simulink model "M_6DoF_BS_Full_backup_11_25_2018"  (R2018a)
settings: Solver=ode4  StartTime=0.0  StopTime=80  FixedStep=0.01  RelTol=1e-3  EnableMultiTasking=on
values from neighbouring files (symbols this model uses):
  b = 1.5652e-08 * (60/(2*pi))^2    (= 1.42729124973e-06)    [Main_run.m]    (also in golden_search.m = x2)
  cbar = 0.04    [Main_run.m]
  Cd = 0.001    [Main_run.m]
  deltaT = 15    [Main_run.m]
  g = 9.81    [Main_run.m]
  Gama1 = diag([3,3,3])    [Main_run.m]
  Gama2 = diag([0.1,0.1,0.1])    [Main_run.m]
  I_B = diag([Ix,Iy,Iz])    [Main_run.m]
  I_r = 3.357e-5    (= 3.357e-05)    [Main_run.m]
  InitialEulerAngles = [psi_i,theta_i,phi_i]    [Main_run.m]
  k = 2.0862e-10 * (60/(2*pi))^2    (= 1.90238627983e-08)    [Main_run.m]    (also in golden_search.m = 2)
  Kd = diag([2,2,2])    [Main_run.m]
  Ki = diag([0.01,0.01,0.01])    [Main_run.m]
  Kp = diag([1,1,1])    [Main_run.m]
  l = 0.225    [Main_run.m]    (also in try1.m = nb * trapz(psi, cl * 0.5 .* rho .* (vt*u).^2 .*c2 , 2) / (2*; try2.m = nb * trapz(psi, cl * 0.5 .* rho .* (vt*u).^2 .*c2 , 2) / (2*)
  Lambda = diag([10,10,10])    [Main_run.m]
  m = 1.035 * 4/6    (= 0.69)    [Main_run.m]
  Omega_i = [0;0;0]    [Main_run.m]
  r = linspace(floor(nr*0.01)/nr,1,nr)    [Main_run.m]    (also in Propeller.m = geometry(10,1:nr); try1.m = geometry(10,1:nr); try2.m = geometry(10,1:nr))
  R_i = [0.0;0.0;0.0]    [Main_run.m]
  t_phase3 = 10    [Main_run.m]
  Tbar = diag([15,15,15])    [Main_run.m]
  tf_phase1 = 10    [Main_run.m]
  tf_phase2 = tf_phase1 + length_phase2*60    (= 70)    [Main_run.m]
  V_i = [0.0;0.0;-0.001]    [Main_run.m]
  Wind_dir = 30 + 180    (= 210)    [Main_run.m]
  xdot_cruise = 15    [Main_run.m]
  zf_phase1 = -40    [Main_run.m]
undefined symbols (not defined in the file or in its folder): eul_0, HDBK, MIL, Moderate, wind_table, wind_time
libraries: sharedtransform x6, aerolibconvert2 x3, aerolibwind2 x3, sharedutil x2, simulink x1, aerolibutil x1, dspmathops x1
(part 2 of 2)

== matlab function M_6DoF_BS_Full_backup_11_25_2018/MATLAB Function1 ==
  settings: updateMethod=DISCRETE
  data: rpm_guesses input; RPM output; RPM2 output; V_rel_B input; angles input; t input; k input; b input; Tau_initial output; T_final output; Tau_final output; l input; geometry data_store_memory
function [RPM,RPM2,Tau_initial,T_final,Tau_final] = FWF(rpm_guesses,V_rel_B,angles,t,k,b,l)
%#codegen

% governing equations

% T=T1+T2+T3+T4 ;
% TA1=l*(T4-T2) ;   roll positive right wing down
% TA2=l*(T1-T3) ;    pitch up positive
% TA3=ta1+ta2+ta3+ta4 ;

% it looks like in atitude control output of the functin should be pitch
% down positive

%%
% predefining vriables for Codegen

T_final=0;
Tau_initial=zeros(3,1);
Tau_final=zeros(3,1);
T2=zeros(4,1);

TA=zeros(3,1);
TA1=zeros(4,1);
TA2=zeros(4,1);
TA3=zeros(4,1);
ta1=zeros(4,1);
ta2=zeros(4,1);
ta3=zeros(4,1);

RPM2=zeros(4,1);
RPM=zeros(4,1);


T = b * rpm_guesses.^2; % requested thrust from rotor r
Tau = k * rpm_guesses.^2;     % requested torques from rotor r

for i=1:4
    % optimization to find optimum rpm where both momentum annd blade element theories match
    
    subfcn2 = @(rpm) try1(rpm,V_rel_B,T(i),angles);
    
    rpm=golden_search(100,16000,subfcn2);
    
    [~,roll,pitch,yaw]=try1(rpm,V_rel_B,T(i),angles);
    
    % rpm to rad/second
    RPM(i)=rpm*2*pi/60;
    
    % torques of a rotor - rotor 1 is the leading edge rotor,left
    % number 2, right number 4, aft number
    
    ta1(i) = roll * (-1)^(i);
    ta2(i) = pitch * (-1)^(i+1);
    ta3(i) = yaw * (-1)^(i+1);
    
end

Tau_initial=[sum(ta1);sum(ta2);sum(ta3)];

%% new addition to help with yaw moment

% here we need to find a way to chage RPMs a bit such that they also
% provide the required Ta3. So, we can find the thrust and torque
% coefficients for a specific time and flight condition.

bb=T./RPM.^2;
kk=Tau./RPM.^2;

M=[bb'; ...
    0,bb(2)*l,0,-bb(4)*l;...
    bb(1)*l,0,-bb(3)*l,0;...
    kk(1),-kk(2),kk(3),-kk(4)];

T_tot=sum(T);

% we use the requsted thrust and torque - here we used the actual
% conventions, down pos z, right wing pos y, pointing to nose pos x

TA(1) = l* (T(2)-T(4)) - Tau_initial(1); % roll
TA(2) = l* (T(1)-T(3)) - Tau_initial(2); % pitch
TA(3) = dot([k,-k,k,-k],rpm_guesses.^2'); %yaw

% newly obtained RPMs
RPM2=(M\[T_tot;TA(1);TA(2);TA(3)]).^0.5;

% now let's see how much thrust and torque they make

for i=1:4
    % input to propeller code must be RPM not rev/sec
    
    subfcn2 = @(T) try2(T,rpm,V_rel_B,angles);
    
    T=golden_search(0,20,subfcn2);
    
    [~,roll,pitch,yaw,T]=try2(T,RPM2(i)*60/(2*pi),V_rel_B,angles);
    
    T2(i)=T;
    TA1(i)=roll* (-1)^(i);
    TA2(i)=pitch* (-1)^(i+1);
    TA3(i)=yaw* (-1)^(i+1);
end

TA_rotor=[sum(TA1);sum(TA2);sum(TA3)];

% here since we don't use negative thrusts, conventions are changed
T_final=sum(T2);
Tau_final(1,1)=l*(T2(2)-T2(4))+TA_rotor(1) ; % roll
Tau_final(2,1)=l*(T2(1)-T2(3))+TA_rotor(2) ; % pitch
Tau_final(3,1)=TA_rotor(3) ;

end

== matlab function M_6DoF_BS_Full_backup_11_25_2018/Aero models/MATLAB Function2 ==
  settings: updateMethod=DISCRETE
  data: rpm_guesses input; RPM output; RPM2 output; V_rel_B input; angles input; t input; k input; b input; Tau_initial output; T_final output; Tau_final output; l input; geometry data_store_memory; power output
%     Copyright (C) 12/12/2018  Regents of the University of Michigan
%     Aerospace Engineering Department
%     Computational Aeroscience Lab, written by Behdad Davoudi

%     This program is free software: you can redistribute it and/or modify
%     it under the terms of the GNU General Public License as published by
%     the Free Software Foundation, either version 3 of the License, or
%     (at your option) any later version.
% 
%     This program is distributed in the hope that it will be useful,
%     but WITHOUT ANY WARRANTY; without even the implied warranty of
%     MERCHANTABILITY or FITNESS FOR A PARTICULAR PURPOSE.  See the
%     GNU General Public License for more details.
% 
%     You should have received a copy of the GNU General Public License
%     along with this program.  If not, see <https://www.gnu.org/licenses/>.

function [RPM,RPM2,Tau_initial,T_final,Tau_final,power] = Radial_inflow(rpm_guesses,V_rel_B,angles,t,k,b,l)
%#codegen

% governing equations

% T=T1+T2+T3+T4 ;
% TA1=l*(T4-T2) ; roll positive right wing down
% TA2=l*(T1-T3) ; pitch up positive
% TA3=ta1+ta2+ta3+ta4 ;
% predefining vriables for Codegen

T_final=0;
Tau_initial=zeros(3,1);
Tau_final=zeros(3,1);
T2=zeros(4,1);

TA=zeros(3,1);
TA1=zeros(4,1);
TA2=zeros(4,1);
TA3=zeros(4,1);
ta1=zeros(4,1);
ta2=zeros(4,1);
ta3=zeros(4,1);
pow=zeros(4,1);

RPM2=zeros(4,1);
RPM=zeros(4,1);


T = b * rpm_guesses.^2;       % requested thrust from rotor r
Tau = k * rpm_guesses.^2;     % requested torques from rotor r


for i=1:4
    
    
    subfcn2 = @(rpm) inv_engine_new(rpm,V_rel_B,T(i));
    
    rpm=golden_search(100,16000,subfcn2);
    
    [~,~,yaw]=inv_engine_new(rpm,V_rel_B,T(i));
    
    % RPM to rad/second
    RPM(i)= rpm*2*pi/60;
    
    ta1(i) = 0;
    ta2(i) = 0;
     % the sign will be taken care of in Matrix M -- no worries!
    ta3(i) = yaw * (+1)^(i+1);
    
    
end

Tau_initial=[sum(ta1);sum(ta2);sum(ta3)];

% end of old way -- there is no control on TA3 that can make the system
% unstable, to do the new way only comment RPM(r) ane let the code keep
% running to the next section

%% new addition to help with yaw moment

% here we need to find a way to chage RPMs a bit such that they also
% provide the required Ta3. So, we can find the thrust and torque
% coefficients for a specific time and flight condition.

bb=T./RPM.^2;
kk=ta3./RPM.^2;

M=[bb'; ...
    0,bb(2)*l,0,-bb(4)*l;...
    bb(1)*l,0,-bb(3)*l,0;...
    kk(1),-kk(2),kk(3),-kk(4)];

T_tot=sum(T);

% we use the requsted thrust and torque - here we used the actual
% conventions, down pos z, right wing pos y, pointing to nose pos x

TA(1) = l* (T(2)-T(4)) - Tau_initial(1); % roll
TA(2) = l* (T(1)-T(3)) - Tau_initial(2); % pitch
TA(3) = dot([k,-k,k,-k],rpm_guesses.^2'); %yaw

% newly obtained RPMs
RPM2=(M\[T_tot;TA(1);TA(2);TA(3)]).^0.5;

% now let's see how much thrust and torque they make

for i=1:4
    % input to propeller code must be RPM not rev/sec
    [T,yaw,p]=Propeller(RPM2(i)*60/(2*pi),V_rel_B);
    
    pow(i)=p;
    T2(i)=T;
    TA1(i)=0;
    TA2(i)=0;
    TA3(i)=yaw* (-1)^(i+1);
    
end

TA_rotor=[sum(TA1);sum(TA2);sum(TA3)];

% here since we don't use negative thrusts, conventions are changed
T_final=sum(T2);
Tau_final(1,1)=l*(T2(2)-T2(4))+TA_rotor(1) ; % roll
Tau_final(2,1)=l*(T2(1)-T2(3))+TA_rotor(2) ; % pitch
Tau_final(3,1)=TA_rotor(3) ;

power = sum(pow) ;

end

== matlab function M_6DoF_BS_Full_backup_11_25_2018/Reference Trajectory2 ==
  data: R_d output; V_d output; t input; psi output; rates_ref output; tf_1 input; zf_1 input; tf_2 input; t_phase3 input; xdot_cruise input; deltaT input; A_d output
%     Copyright (C) 12/12/2018  Regents of the University of Michigan
%     Aerospace Engineering Department
%     Computational Aeroscience Lab, written by Behdad Davoudi

%     This program is free software: you can redistribute it and/or modify
%     it under the terms of the GNU General Public License as published by
%     the Free Software Foundation, either version 3 of the License, or
%     (at your option) any later version.
% 
%     This program is distributed in the hope that it will be useful,
%     but WITHOUT ANY WARRANTY; without even the implied warranty of
%     MERCHANTABILITY or FITNESS FOR A PARTICULAR PURPOSE.  See the
%     GNU General Public License for more details.
% 
%     You should have received a copy of the GNU General Public License
%     along with this program.  If not, see <https://www.gnu.org/licenses/>.

function [R_d, V_d, psi, rates_ref, A_d] = fcn(t, tf_1, zf_1, tf_2, t_phase3, xdot_cruise, deltaT)
%#codegen

x = 0;
y = 0;
z = 0;
xdot = 0;
ydot = 0;
zdot = 0;
xddot=0;
yddot =0;
zddot = 0;

if t<=tf_1
    
    xdot = 0;
    ydot = 0;
    z_f = zf_1;
    tf = tf_1;
    a = -(2*z_f)/tf^3;
    b = (3*z_f)/tf^2;
    z = a*t.^3+b*t.^2;
    zdot = 3*a*t.^2+2*b*t;
    zddot = 6*a*t+2*b;
elseif t>tf_1 && t<=tf_2
    z = zf_1;
    zdot = 0;
    if (t-tf_1)<=deltaT
        xdot = xdot_cruise/deltaT*(t-tf_1);
        x = 0.5*xdot_cruise/deltaT*(t-tf_1)^2;
    elseif (t-tf_1)>deltaT && (t-tf_1)<(tf_2-deltaT)
        xdot = xdot_cruise;
        x = 0.5*deltaT*xdot_cruise + xdot_cruise*(t-tf_1-deltaT); 
    end
    if t>(tf_2-deltaT)
        xdot = xdot_cruise-xdot_cruise/deltaT*(t-(tf_2-deltaT));
        x = 0.5*deltaT*xdot_cruise+xdot_cruise*(tf_2-tf_1-2*deltaT)+0.5*(xdot_cruise+xdot)*(t-(tf_2-deltaT));
    end
    
elseif t>tf_2
    x = deltaT*xdot_cruise+xdot_cruise*(tf_2-tf_1-2*deltaT);
    xdot = 0;
    z_i = zf_1;
    tt = t-tf_2;
    tf = t_phase3;
    a = (2*z_i)/tf^3;
    b = -(3*z_i)/tf^2;
    d = z_i;
    z = a*tt.^3+b*tt.^2+d;
    zdot = 3*a*tt.^2+2*b*tt;
    
end

R_d = [x;y;z];
V_d = [xdot;ydot;zdot];
A_d = [xddot;yddot;zddot];
%psi = sin(2*pi*t/80);
psi =0;
rates_ref = [0;0;0];

end

== matlab function M_6DoF_BS_Full_backup_11_25_2018/Reference Trajectory3 ==
  data: R_d output; V_d output; t input; psi output; rates_ref output; tf_1 input; zf_1 input; tf_2 input; t_phase3 input; xdot_cruise input; deltaT input; A_d output
function [R_d, V_d, psi, rates_ref, A_d] = fcn(t, tf_1, zf_1, tf_2, t_phase3, xdot_cruise, deltaT)
%#codegen

% 500 seconds simulation time is required.

x = 0;
y = 0;
z = 0;
xdot = 0;
ydot = 0;
zdot = 0;
xddot=0;
yddot =0;
zddot = 0;

xdotmax=20;
xdotmin=0;
nmax=20;
% note length of simulation = nmax * (dta+dtc)
xdot_cruise=linspace(xdotmin,xdotmax,nmax);

dtc=20;
dta=5;

n=floor(t/(dtc+dta))+1;

if t== nmax*(dta+dtc)
   n=n-1 ;
end

t2=t-(n-1)*(dtc+dta);

if t2<=dtc
   
  xdot = xdot_cruise(n);  
  x = xdot_cruise(n) * t2;
  
  if n>1
    for i=1:n-1   
        x= 0.5 *  (xdot_cruise(i+1) - xdot_cruise(i)) / dta * dta^2 + xdot_cruise(i) *(dtc+dta) + x  ;
    end
  end
  
elseif t2>dtc && t2<=dtc+dta
    
  xdot = (xdot_cruise(n+1) - xdot_cruise(n))/dta * (t2-dtc) + xdot_cruise(n);  
  
  x = 0.5 * (xdot_cruise(n+1)- xdot_cruise(n)) / dta * (t2-dtc)^2 + xdot_cruise(n) * (t2-dtc) + xdot_cruise(n) * dtc ;
  
  if n>1
    for i=1:n-1   
        x= 0.5 * (xdot_cruise(i+1)- xdot_cruise(i)) / dta * dta^2 + xdot_cruise(i) *(dtc+dta) + x  ;
    end
  end

end

R_d = [x;y;z];
V_d = [xdot;ydot;zdot];
A_d = [xddot;yddot;zddot];
%psi = sin(2*pi*t/80);
psi =0;
rates_ref = [0;0;0];

end
